simulink model "noise"  (R2017b)
settings: Solver=FixedStepAuto  StartTime=0.0  StopTime=1000  FixedStep=0.01  MaxStep=0.01  RelTol=1e-3
values from neighbouring files (symbols this model uses):
  b1 = 1    [test.m]
  b2 = 2    [test.m]
settings Model: Creator=rablanco.ext  LastModifiedBy=rablanco.ext

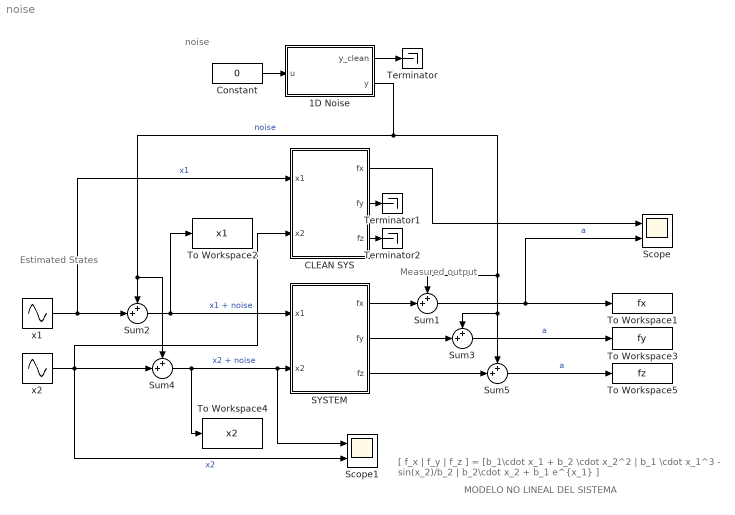
== system noise ==
  note: MODELO NO LINEAL DEL SISTEMA
  note: [ f_x | f_y | f_z ] = [b_1\cdot x_1 + b_2 \cdot x_2^2 | b_1 \cdot x_1^3 - sin(x_2)/b_2 | b_2\cdot x_2 + b_1 e^{x_1} ]
  note: noise
  note: Measured output
  note: Estimated States
  1D Noise : MATLAB Function  TreatAsAtomicUnit=on
  CLEAN SYS : Subsystem
  Constant : Constant  Value=0
  SYSTEM : Subsystem
  Scope : Scope  NumInputPorts=2
  Scope1 : Scope  NumInputPorts=2
  Sum{1..5} (5 alike) : Sum  Inputs=++|
  Terminator : Terminator
  Terminator1 : Terminator
  Terminator2 : Terminator
  To Workspace1 : ToWorkspace  VariableName=fx  SampleTime=-1
  To Workspace2 : ToWorkspace  VariableName=x1  SampleTime=-1
  To Workspace3 : ToWorkspace  VariableName=fy  SampleTime=-1
  To Workspace4 : ToWorkspace  VariableName=x2  SampleTime=-1
  To Workspace5 : ToWorkspace  VariableName=fz  SampleTime=-1
  x1 : Sin  SampleTime=0
  x2 : Sin  SampleTime=0
  wires:
  1D Noise/1(y_clean) -> Terminator/1
  Constant/1 -> 1D Noise/1(u)
  Sum1/1 -> To Workspace1/1, Scope/2  "a"
  Sum3/1 -> To Workspace3/1  "a"
  Sum5/1 -> To Workspace5/1  "a"
  1D Noise/2(y) -> Sum1/1, Sum3/1, Sum5/1, Sum4/1, Sum2/1  "noise"
  x2/1 -> Scope1/2, Sum4/2, CLEAN SYS/2(x2)  "x2"
  x1/1 -> Sum2/2, CLEAN SYS/1(x1)  "x1"
  SYSTEM/1(fx) -> Sum1/2
  SYSTEM/2(fy) -> Sum3/2
  SYSTEM/3(fz) -> Sum5/2
  CLEAN SYS/1(fx) -> Scope/1
  CLEAN SYS/2(fy) -> Terminator1/1
  CLEAN SYS/3(fz) -> Terminator2/1
  Sum2/1 -> SYSTEM/1(x1), To Workspace2/1  "x1 + noise"
  Sum4/1 -> To Workspace4/1, Scope1/1, SYSTEM/2(x2)  "x2 + noise"

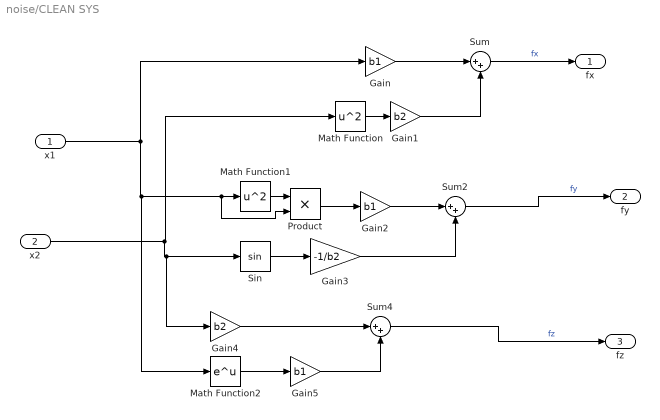
== system noise/CLEAN SYS ==
  x1 : Inport
  x2 : Inport  Port=2
  Gain : Gain  Gain=b1
  Gain1 : Gain  Gain=b2
  Gain2 : Gain  Gain=b1
  Gain3 : Gain  Gain=-1/b2
  Gain4 : Gain  Gain=b2
  Gain5 : Gain  Gain=b1
  Math Function : Math  Operator=square  SaturateOnIntegerOverflow=on
  Math Function1 : Math  Operator=square  SaturateOnIntegerOverflow=on
  Math Function2 : Math  SaturateOnIntegerOverflow=on
  Product : Product
  Sin : Trigonometry
  Sum : Sum  Inputs=|++
  Sum2 : Sum  Inputs=|++
  Sum4 : Sum  Inputs=|++
  fx : Outport
  fy : Outport  Port=2
  fz : Outport  Port=3
  wires:
  x1/1 -> Math Function2/1, Product/2, Math Function1/1, Gain/1
  x2/1 -> Gain4/1, Sin/1, Math Function/1
  Sum/1 -> fx/1  "fx"
  Sum2/1 -> fy/1  "fy"
  Sum4/1 -> fz/1  "fz"
  Product/1 -> Gain2/1
  Math Function/1 -> Gain1/1
  Math Function1/1 -> Product/1
  Math Function2/1 -> Gain5/1
  Gain/1 -> Sum/1
  Gain1/1 -> Sum/2
  Gain4/1 -> Sum4/1
  Gain5/1 -> Sum4/2
  Sin/1 -> Gain3/1
  Gain2/1 -> Sum2/1
  Gain3/1 -> Sum2/2

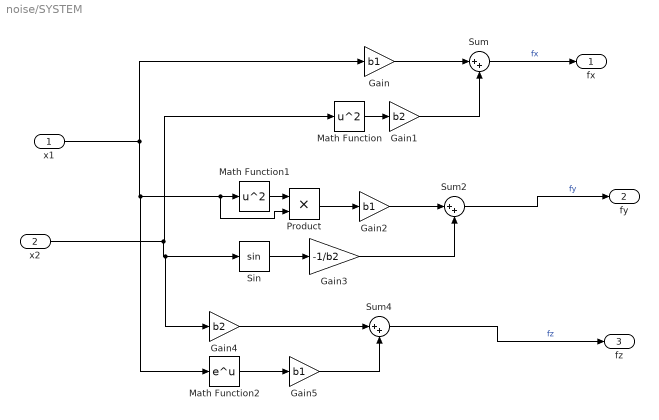
== system noise/SYSTEM ==
  x1 : Inport
  x2 : Inport  Port=2
  Gain : Gain  Gain=b1
  Gain1 : Gain  Gain=b2
  Gain2 : Gain  Gain=b1
  Gain3 : Gain  Gain=-1/b2
  Gain4 : Gain  Gain=b2
  Gain5 : Gain  Gain=b1
  Math Function : Math  Operator=square  SaturateOnIntegerOverflow=on
  Math Function1 : Math  Operator=square  SaturateOnIntegerOverflow=on
  Math Function2 : Math  SaturateOnIntegerOverflow=on
  Product : Product
  Sin : Trigonometry
  Sum : Sum  Inputs=|++
  Sum2 : Sum  Inputs=|++
  Sum4 : Sum  Inputs=|++
  fx : Outport
  fy : Outport  Port=2
  fz : Outport  Port=3
  wires:
  x1/1 -> Math Function2/1, Product/2, Math Function1/1, Gain/1
  x2/1 -> Gain4/1, Sin/1, Math Function/1
  Sum/1 -> fx/1  "fx"
  Sum2/1 -> fy/1  "fy"
  Sum4/1 -> fz/1  "fz"
  Product/1 -> Gain2/1
  Math Function/1 -> Gain1/1
  Math Function1/1 -> Product/1
  Math Function2/1 -> Gain5/1
  Gain/1 -> Sum/1
  Gain1/1 -> Sum/2
  Gain4/1 -> Sum4/1
  Gain5/1 -> Sum4/2
  Sin/1 -> Gain3/1
  Gain2/1 -> Sum2/1
  Gain3/1 -> Sum2/2

== matlab function noise/1D Noise ==
  data: y_clean output; u input; y output
function [y_clean,y] = fcn(u)
y_clean = u;
max_u=1;
noise = max_u.*.5.*(-1+2.*rand(1)); % rand num (-1,1)*(25% of u)->(-25%,25%) of u
y = u+ noise;
